simulink model "Sistema"  (R2021b)
settings: Solver=ode15s  StartTime=0.0  StopTime=10.0  MaxStep=1E-3  RelTol=1e-3
libraries: fl_lib x14, nesl_utility x6, slpidlib x1
settings Model: Creator=lunit  LastModifiedBy=lunit
settings DataIOCC: SaveFormat=Array  ReturnWorkspaceOutputs=off  TimeSaveName=t
settings DebuggingCC: AlgebraicLoopMsg=none  ArtificialAlgebraicLoopMsg=none  MaxConsecutiveZCsMsg=none  ModelReferenceExtraNoncontSigs=none  OperatingPointInterfaceChecksumMismatchMsg=none

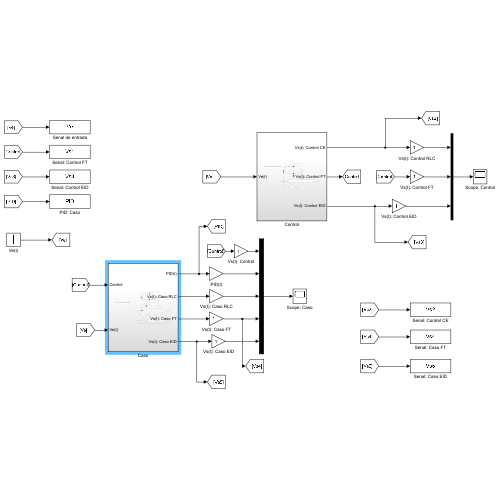
[thumbnail: Simulink's stored preview of the top-level diagram]
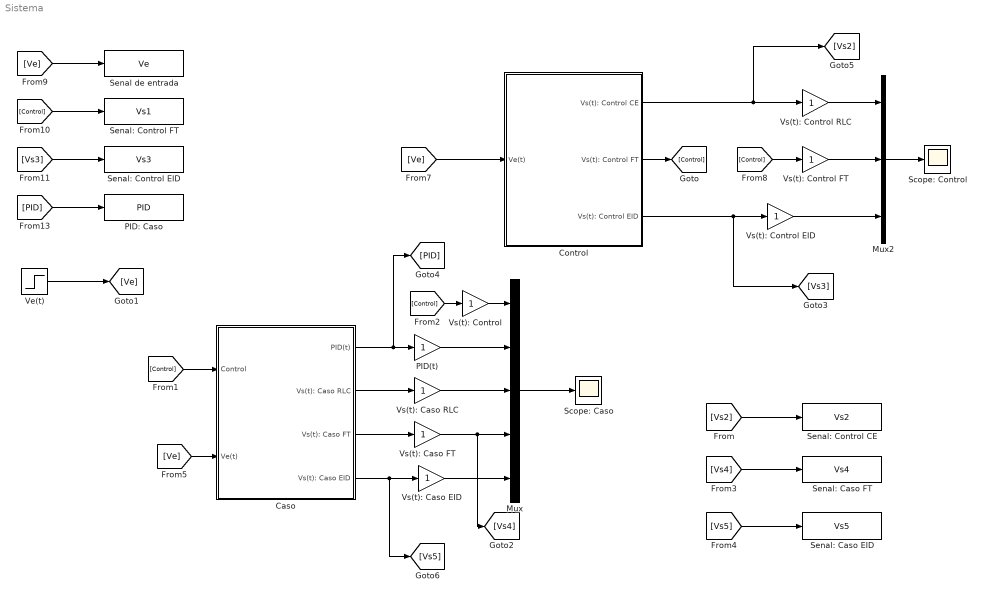
== system Sistema ==
  Caso : Subsystem
  Control : Subsystem
  Mux : Mux  Inputs=5
  Mux2 : Mux  Inputs=3
  PID(t) : Gain
  PID: Caso : ToWorkspace  VariableName=PID  SampleTime=-1
  Scope: Caso : Scope
  Scope: Control : Scope
  Senal de entrada : ToWorkspace  VariableName=Ve  SampleTime=-1
  Senal: Caso EID : ToWorkspace  VariableName=Vs5  SampleTime=-1
  Senal: Caso FT : ToWorkspace  VariableName=Vs4  SampleTime=-1
  Senal: Control CE : ToWorkspace  VariableName=Vs2  SampleTime=-1
  Senal: Control EID : ToWorkspace  VariableName=Vs3  SampleTime=-1
  Senal: Control FT : ToWorkspace  VariableName=Vs1  SampleTime=-1
  Ve(t) : Step  Time=0  Before=1  SampleTime=0
  Vs(t): Caso EID : Gain
  Vs(t): Caso FT : Gain
  Vs(t): Caso RLC : Gain
  Vs(t): Control : Gain
  Vs(t): Control EID : Gain
  Vs(t): Control FT : Gain
  Vs(t): Control RLC : Gain
  wires:
  [Control] -> Caso/1(Control)
  Control/2(Vs(t): Control FT) -> [Control]
  [Ve] -> Control/1(Ve(t))
  Mux2/1 -> Scope: Control/1
  Control/1(Vs(t): Control CE) -> Vs(t): Control RLC/1, [Vs2]
  [Control] -> Vs(t): Control FT/1
  [Ve] -> Senal de entrada/1
  [Control] -> Senal: Control FT/1
  [Vs3] -> Senal: Control EID/1
  [PID] -> PID: Caso/1
  Ve(t)/1 -> [Ve]
  Vs(t): Control FT/1 -> Mux2/2
  Vs(t): Control RLC/1 -> Mux2/1
  [Control] -> Vs(t): Control/1
  Caso/1(PID(t)) -> PID(t)/1, [PID]
  PID(t)/1 -> Mux/2
  Vs(t): Caso RLC/1 -> Mux/3
  Vs(t): Caso FT/1 -> [Vs4], Mux/4
  [Vs2] -> Senal: Control CE/1
  Caso/2(Vs(t): Caso RLC) -> Vs(t): Caso RLC/1
  Caso/3(Vs(t): Caso FT) -> Vs(t): Caso FT/1
  [Ve] -> Caso/2(Ve(t))
  Mux/1 -> Scope: Caso/1
  Control/3(Vs(t): Control EID) -> [Vs3], Vs(t): Control EID/1
  Vs(t): Control EID/1 -> Mux2/3
  [Vs4] -> Senal: Caso FT/1
  Caso/4(Vs(t): Caso EID) -> [Vs5], Vs(t): Caso EID/1
  [Vs5] -> Senal: Caso EID/1
  Vs(t): Control/1 -> Mux/1
  Vs(t): Caso EID/1 -> Mux/5

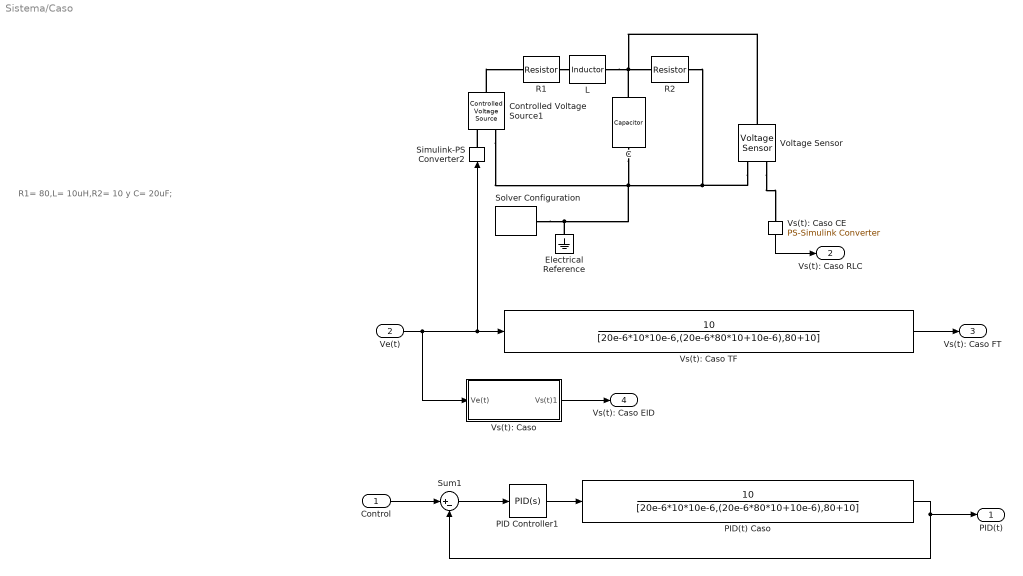
== system Sistema/Caso ==
  note: R1= 80,L= 10uH,R2= 10 y C= 20uF;
  Control : Inport
  Ve(t) : Inport  Port=2
  C : fl_lib/Electrical/Electrical Elements/Capacitor  c=20 uF  r=1e-6 Ohm  g=0 1/Ohm  i_specify=off  i_priority=None  i=0 A  i_nominal_specify=off  i_nominal_unit=A  i_nominal_value=1  v_specify=off  v_priority=None  v=0 V  v_nominal_specify=off  v_nominal_unit=V  v_nominal_value=1  vc_specify=off  vc_priority=High  vc=0 V  vc_nominal_specify=off  vc_nominal_unit=V  vc_nominal_value=1
  Controlled Voltage Source1 : fl_lib/Electrical/Electrical Sources/Controlled Voltage Source
  Electrical Reference : fl_lib/Electrical/Electrical Elements/Electrical Reference
  L : fl_lib/Electrical/Electrical Elements/Inductor  l=10 uH  r=0 Ohm  g=1e-9 1/Ohm  i_specify=off  i_priority=None  i=0 A  i_nominal_specify=off  i_nominal_unit=A  i_nominal_value=1  v_specify=off  v_priority=None  v=0 V  v_nominal_specify=off  v_nominal_unit=V  v_nominal_value=1  i_L_specify=off  i_L_priority=High  i_L=0 A  i_L_nominal_specify=off  i_L_nominal_unit=A  i_L_nominal_value=1
  PID Controller1 : slpidlib/PID Controller  Controller=PID  Form=Parallel  TimeDomain=Continuous-time  UseExternalTs=off  SampleTime=-1  IntegratorMethod=Forward Euler  FilterMethod=Forward Euler  ControllerParametersSource=internal  P=0.576682613237128  I=3241.80421910214  D=0  UseFilter=on  N=100  TunerSelectOption=Transfer Function Based (PID Tuner App)  InitialConditionSource=internal  InitialConditionForIntegrator=0  InitialConditionForFilter=0  DifferentiatorICPrevScaledInput=0  ExternalReset=none  TrackingMode=off  Kt=1  LimitOutput=off  SatLimitsSource=internal  UpperSaturationLimit=inf  LowerSaturationLimit=-inf  LinearizeAsGain=on  AntiWindupMode=none  Kb=1  POutMin=[]  POutMax=[]  IOutMin=[]  IOutMax=[]  DOutMin=[]  DOutMax=[]  NOutMin=[]  NOutMax=[]  SumOutMin=[]  SumOutMax=[]  SaturationOutMin=[]  SaturationOutMax=[]  PParamMin=[]  PParamMax=[]  IParamMin=[]  IParamMax=[]  DParamMin=[]  DParamMax=[]  NParamMin=[]  NParamMax=[]  KbParamMin=[]  KbParamMax=[]  KtParamMin=[]  KtParamMax=[]  KbOutMin=[]  KbOutMax=[]  KtOutMin=[]  KtOutMax=[]  IntegratorOutMin=[]  IntegratorOutMax=[]  FilterOutMin=[]  FilterOutMax=[]  SumI1OutMin=[]  SumI1OutMax=[]  SumI2OutMin=[]  SumI2OutMax=[]  SumI3OutMin=[]  SumI3OutMax=[]  SumI4OutMin=[]  SumI4OutMax=[]  SumDOutMin=[]  SumDOutMax=[]  DifferentiatorOutMin=[]  DifferentiatorOutMax=[]  FilterDiffOutCoefMin=[]  FilterDiffOutCoefMax=[]  ReciprocalOutMin=[]  ReciprocalOutMax=[]  SumDenOutMin=[]  SumDenOutMax=[]  SumNumOutMin=[]  SumNumOutMax=[]  DivideOutMin=[]  DivideOutMax=[]  UdiffTsProdOutMin=[]  UdiffTsProdOutMax=[]  NTsProdOutMin=[]  NTsProdOutMax=[]  UintegralTsProdOutMin=[]  UintegralTsProdOutMax=[]  UngainTsProdOutMin=[]  UngainTsProdOutMax=[]  IntegratorContinuousStateAttributes=''  IntegratorStateMustResolveToSignalObject=off  IntegratorRTWStateStorageClass=Auto  FilterContinuousStateAttributes=''  FilterStateMustResolveToSignalObject=off  FilterRTWStateStorageClass=Auto  ParallelPVariant=InternalParameters  IdealPVariant=Disabled  IVariant=InternalParameters  DVariant=InternalParameters  IntegratorVariant=Continuous  SatVariant=Disabled  AWVariant=Passthrough  PCopyVariant=Disabled  TRVariant=Disabled  FdbkBlocksVariant=Forward  IdealPFdbkVariant=Disabled  SatFdbkVariant=Disabled  DerivativeFilterVariant=ContFilter  NVariant=InternalParameters  NCopyVariant=Disabled  FilterICVariant=InternalICsFilter  IntegratorICVariant=InternalICs  ExternalResetVariant=Disabled  TRSumVariant=Passthrough  SumFdbkVariant=Disabled  SumVariant=Sum_PID  TsampFilterVariant=InternalTs  TsampNgainVariant=Passthrough  TsampIntegralVariant=Passthrough  ExternalSaturationOutDataTypeStr=Inherit: Same as second input
  PID(t) Caso : TransferFcn  Numerator=[10]  Denominator=[20e-6*10*10e-6,(20e-6*80*10+10e-6),80+10]
  R1 : fl_lib/Electrical/Electrical Elements/Resistor  R=80 Ohm  i_specify=off  i_priority=None  i=0 A  i_nominal_specify=off  i_nominal_unit=A  i_nominal_value=1  v_specify=off  v_priority=None  v=0 V  v_nominal_specify=off  v_nominal_unit=V  v_nominal_value=1
  R2 : fl_lib/Electrical/Electrical Elements/Resistor  R=10 Ohm  i_specify=off  i_priority=None  i=0 A  i_nominal_specify=off  i_nominal_unit=A  i_nominal_value=1  v_specify=off  v_priority=None  v=0 V  v_nominal_specify=off  v_nominal_unit=V  v_nominal_value=1
  Simulink-PS Converter2 : nesl_utility/Simulink-PS Converter  PhysicalDomain=network_engine_domain  SubClassName=ps_input  LeftPortType=input  RightPortType=output  PseudoPeriodic=off  Frequencies=[]  NoiseDistribution=none  NoiseParameters=[]  Unit=1  AffineConversion=off  FilteringAndDerivatives=provide  SimscapeFilterOrder=1  InputFilterTimeConstant=0.001  UdotUserProvided=0
      settings: SourceProductBaseCode=PW,SS
  Solver Configuration : nesl_utility/Solver Configuration  PhysicalDomain=network_engine_domain  SubClassName=solver  LeftPortType=input  RightPortType=generic  Tones=[]  Harmonics=[]  SimulateNoise=off  Profile=off  UseLocalSampling=off  EnableSwitchedLinearOptims=on  FrequencyDomain=off  UseCCode=off  RelTol=0.001  AbsTol=1e-06  MinStep=1e-09  ToWorkspace=off  RevertToSquareIcSolve=off  NumHomotopyIterations=100  PhasorMode=off  PhasorModeNumHarmonics=1  DoDC=off  ResidualTolerance=1e-09  UseLocalSolver=off  LocalSolverChoice=NE_BACKWARD_EULER_ADVANCER  LocalSolverSampleTime=0.001  DoFixedCost=off  MaxNonlinIter=3  MaxModeIter=2  ComputeImpulses=off  ImpulseIterations=2  LinearAlgebra=auto  EquationFormulation=NE_TIME_EF  DelaysMemoryBudget=1024  AutomaticFiltering=on  FilteringTimeConstant=0.001  PartitionStorageMethod=AS_NEEDED  PartitionMemoryBudget=1024  PartitionMethod=ROBUST
      settings: SourceProductBaseCode=PW,SS
  Sum1 : Sum  Inputs=|+-
  Voltage Sensor : fl_lib/Electrical/Electrical Sensors/Voltage Sensor
  Vs(t): Caso : Subsystem
  Vs(t): Caso CE : nesl_utility/PS-Simulink Converter  PhysicalDomain=network_engine_domain  SubClassName=ps_output  LeftPortType=input  RightPortType=output  PseudoPeriodic=off  Frequencies=[]  Unit=inherit  AffineConversion=off
      settings: SourceProductBaseCode=PW,SS
  Vs(t): Caso TF : TransferFcn  Numerator=[10]  Denominator=[20e-6*10*10e-6,(20e-6*80*10+10e-6),80+10]
  PID(t) : Outport
  Vs(t): Caso RLC : Outport  Port=2
  Vs(t): Caso FT : Outport  Port=3
  Vs(t): Caso EID : Outport  Port=4
  wires:
  Sum1/1 -> PID Controller1/1
  PID(t) Caso/1 -> PID(t)/1, Sum1/2
  Control/1 -> Sum1/1
  PID Controller1/1 -> PID(t) Caso/1
  Vs(t): Caso TF/1 -> Vs(t): Caso FT/1
  Vs(t): Caso CE/1 -> Vs(t): Caso RLC/1
  Vs(t): Caso/1(Vs(t)1) -> Vs(t): Caso EID/1
  Ve(t)/1 -> Vs(t): Caso/1(Ve(t)), Simulink-PS Converter2/1, Vs(t): Caso TF/1
  connections:
  Electrical Reference/LConn1 -- Controlled Voltage Source1/RConn2 -- C/RConn1 -- R2/RConn1 -- Voltage Sensor/RConn2 -- Solver Configuration/RConn1
  C/LConn1 -- Voltage Sensor/LConn1 -- L/RConn1 -- R2/LConn1
  R1/RConn1 -- L/LConn1
  Voltage Sensor/RConn1 -- Vs(t): Caso CE/LConn1
  Simulink-PS Converter2/RConn1 -- Controlled Voltage Source1/RConn1
  Controlled Voltage Source1/LConn1 -- R1/LConn1

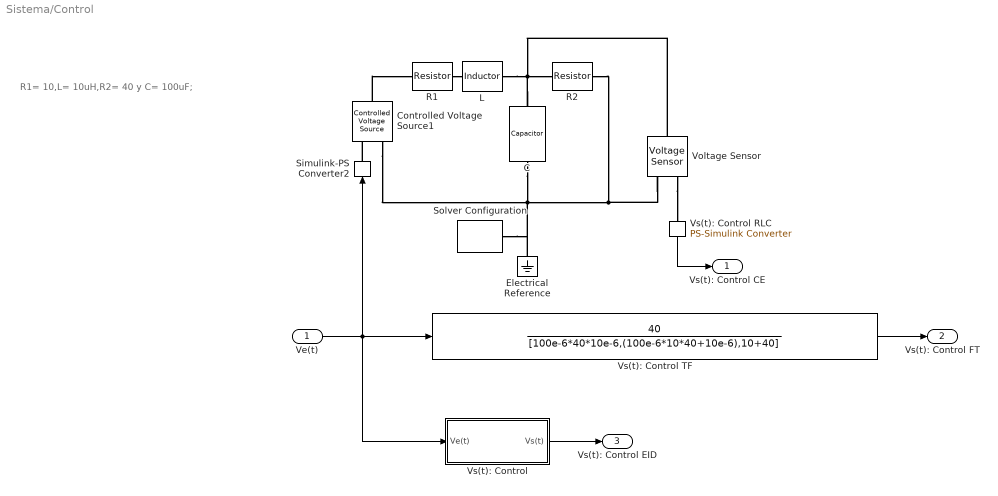
== system Sistema/Control ==
  note: R1= 10,L= 10uH,R2= 40 y C= 100uF;
  Ve(t) : Inport
  C : fl_lib/Electrical/Electrical Elements/Capacitor  c=100 uF  r=1e-6 Ohm  g=0 1/Ohm  i_specify=off  i_priority=None  i=0 A  i_nominal_specify=off  i_nominal_unit=A  i_nominal_value=1  v_specify=off  v_priority=None  v=0 V  v_nominal_specify=off  v_nominal_unit=V  v_nominal_value=1  vc_specify=off  vc_priority=High  vc=0 V  vc_nominal_specify=off  vc_nominal_unit=V  vc_nominal_value=1
  Controlled Voltage Source1 : fl_lib/Electrical/Electrical Sources/Controlled Voltage Source
  Electrical Reference : fl_lib/Electrical/Electrical Elements/Electrical Reference
  L : fl_lib/Electrical/Electrical Elements/Inductor  l=10 uH  r=0 Ohm  g=1e-9 1/Ohm  i_specify=off  i_priority=None  i=0 A  i_nominal_specify=off  i_nominal_unit=A  i_nominal_value=1  v_specify=off  v_priority=None  v=0 V  v_nominal_specify=off  v_nominal_unit=V  v_nominal_value=1  i_L_specify=off  i_L_priority=High  i_L=0 A  i_L_nominal_specify=off  i_L_nominal_unit=A  i_L_nominal_value=1
  R1 : fl_lib/Electrical/Electrical Elements/Resistor  R=10 Ohm  i_specify=off  i_priority=None  i=0 A  i_nominal_specify=off  i_nominal_unit=A  i_nominal_value=1  v_specify=off  v_priority=None  v=0 V  v_nominal_specify=off  v_nominal_unit=V  v_nominal_value=1
  R2 : fl_lib/Electrical/Electrical Elements/Resistor  R=40 Ohm  i_specify=off  i_priority=None  i=0 A  i_nominal_specify=off  i_nominal_unit=A  i_nominal_value=1  v_specify=off  v_priority=None  v=0 V  v_nominal_specify=off  v_nominal_unit=V  v_nominal_value=1
  Simulink-PS Converter2 : nesl_utility/Simulink-PS Converter  PhysicalDomain=network_engine_domain  SubClassName=ps_input  LeftPortType=input  RightPortType=output  PseudoPeriodic=off  Frequencies=[]  NoiseDistribution=none  NoiseParameters=[]  Unit=1  AffineConversion=off  FilteringAndDerivatives=provide  SimscapeFilterOrder=1  InputFilterTimeConstant=0.001  UdotUserProvided=0
      settings: SourceProductBaseCode=PW,SS
  Solver Configuration : nesl_utility/Solver Configuration  PhysicalDomain=network_engine_domain  SubClassName=solver  LeftPortType=input  RightPortType=generic  Tones=[]  Harmonics=[]  SimulateNoise=off  Profile=off  UseLocalSampling=off  EnableSwitchedLinearOptims=on  FrequencyDomain=off  UseCCode=off  RelTol=0.001  AbsTol=1e-06  MinStep=1e-09  ToWorkspace=off  RevertToSquareIcSolve=off  NumHomotopyIterations=100  PhasorMode=off  PhasorModeNumHarmonics=1  DoDC=off  ResidualTolerance=1e-09  UseLocalSolver=off  LocalSolverChoice=NE_BACKWARD_EULER_ADVANCER  LocalSolverSampleTime=0.001  DoFixedCost=off  MaxNonlinIter=3  MaxModeIter=2  ComputeImpulses=off  ImpulseIterations=2  LinearAlgebra=auto  EquationFormulation=NE_TIME_EF  DelaysMemoryBudget=1024  AutomaticFiltering=on  FilteringTimeConstant=0.001  PartitionStorageMethod=AS_NEEDED  PartitionMemoryBudget=1024  PartitionMethod=ROBUST
      settings: SourceProductBaseCode=PW,SS
  Voltage Sensor : fl_lib/Electrical/Electrical Sensors/Voltage Sensor
  Vs(t): Control : Subsystem
  Vs(t): Control RLC : nesl_utility/PS-Simulink Converter  PhysicalDomain=network_engine_domain  SubClassName=ps_output  LeftPortType=input  RightPortType=output  PseudoPeriodic=off  Frequencies=[]  Unit=inherit  AffineConversion=off
      settings: SourceProductBaseCode=PW,SS
  Vs(t): Control TF : TransferFcn  Numerator=[40]  Denominator=[100e-6*40*10e-6,(100e-6*10*40+10e-6),10+40]
  Vs(t): Control CE : Outport
  Vs(t): Control FT : Outport  Port=2
  Vs(t): Control EID : Outport  Port=3
  wires:
  Ve(t)/1 -> Simulink-PS Converter2/1, Vs(t): Control/1(Ve(t)), Vs(t): Control TF/1
  Vs(t): Control RLC/1 -> Vs(t): Control CE/1
  Vs(t): Control TF/1 -> Vs(t): Control FT/1
  Vs(t): Control/1(Vs(t)) -> Vs(t): Control EID/1
  connections:
  Voltage Sensor/RConn1 -- Vs(t): Control RLC/LConn1
  Simulink-PS Converter2/RConn1 -- Controlled Voltage Source1/RConn1
  C/LConn1 -- Voltage Sensor/LConn1 -- L/RConn1 -- R2/LConn1
  R2/RConn1 -- Controlled Voltage Source1/RConn2 -- Electrical Reference/LConn1 -- Solver Configuration/RConn1 -- C/RConn1 -- Voltage Sensor/RConn2
  Controlled Voltage Source1/LConn1 -- R1/LConn1
  R1/RConn1 -- L/LConn1

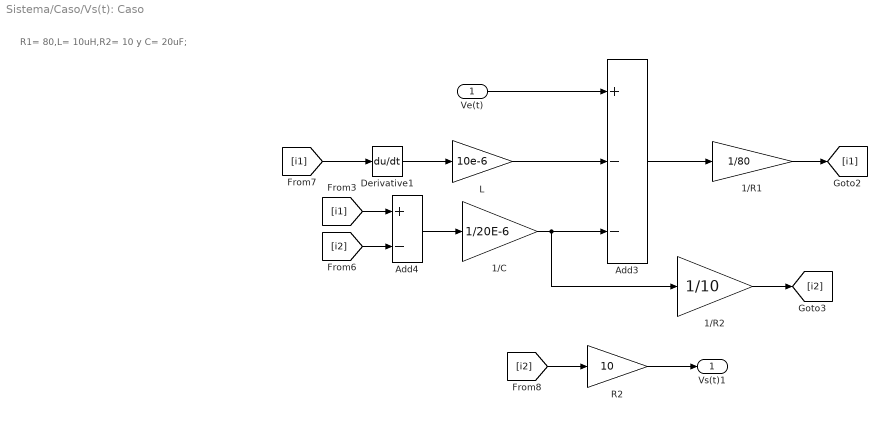
== system Sistema/Caso/Vs(t): Caso ==
  note: R1= 80,L= 10uH,R2= 10 y C= 20uF;
  Ve(t) : Inport
  1/C : Gain  Gain=1/20E-6
  1/R1 : Gain  Gain=1/80
  1/R2 : Gain  Gain=1/10
  Add3 : Sum  Inputs=+--
  Add4 : Sum  Inputs=+-
  Derivative1 : Derivative
  L : Gain  Gain=10e-6
  R2 : Gain  Gain=10
  Vs(t)1 : Outport
  wires:
  [i2] -> Add4/2
  1/C/1 -> 1/R2/1, Add3/3
  Add4/1 -> 1/C/1
  Ve(t)/1 -> Add3/1
  Add3/1 -> 1/R1/1
  1/R2/1 -> [i2]
  Derivative1/1 -> L/1
  [i1] -> Derivative1/1
  [i2] -> R2/1
  L/1 -> Add3/2
  1/R1/1 -> [i1]
  [i1] -> Add4/1
  R2/1 -> Vs(t)1/1

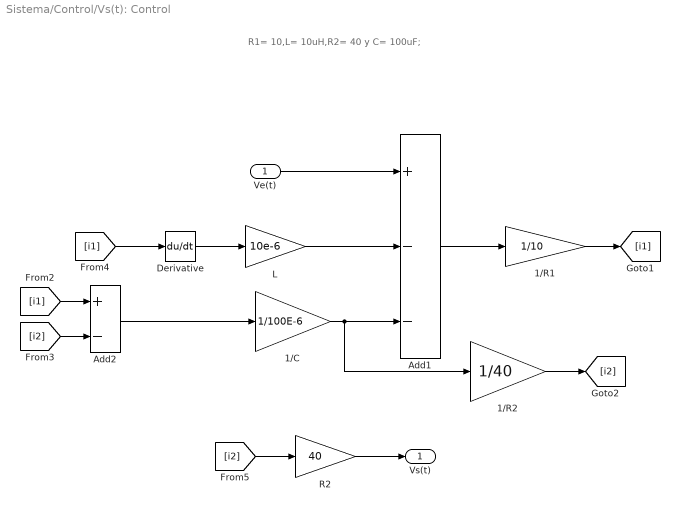
== system Sistema/Control/Vs(t): Control ==
  note: R1= 10,L= 10uH,R2= 40 y C= 100uF;
  Ve(t) : Inport
  1/C : Gain  Gain=1/100E-6
  1/R1 : Gain  Gain=1/10
  1/R2 : Gain  Gain=1/40
  Add1 : Sum  Inputs=+--
  Add2 : Sum  Inputs=+-
  Derivative : Derivative
  L : Gain  Gain=10e-6
  R2 : Gain  Gain=40
  Vs(t) : Outport
  wires:
  Add1/1 -> 1/R1/1
  1/R1/1 -> [i1]
  Derivative/1 -> L/1
  L/1 -> Add1/2
  [i2] -> R2/1
  R2/1 -> Vs(t)/1
  [i1] -> Derivative/1
  Ve(t)/1 -> Add1/1
  1/C/1 -> 1/R2/1, Add1/3
  Add2/1 -> 1/C/1
  [i1] -> Add2/1
  [i2] -> Add2/2
  1/R2/1 -> [i2]
